simulink model "sim_Motor_2kW_openloop_v3_delay"  (Simulink 7.9)
settings: Solver=ode45  StartTime=0.0  StopTime=0.08  RelTol=1e-3
libraries: powerlib x7, simulink_extras x2
settings Model: Creator=Kun Zhang  LastModifiedBy=LYN
settings SolverCC: AutoInsertRateTranBlk=on
settings DebuggingCC: MultiTaskDSMMsg=warning  MultiTaskCondExecSysMsg=none  StrictBusMsg=None
settings RTWCC: IncludeERTFirstTime=on
settings GRTTargetCC: CombineOutputUpdateFcns=off  GRTInterface=on

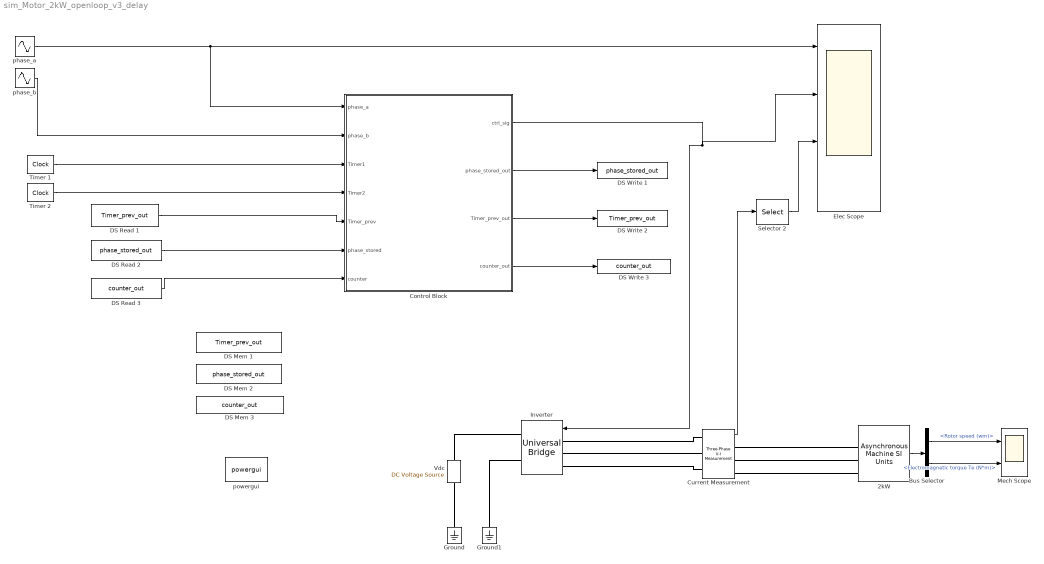
== system sim_Motor_2kW_openloop_v3_delay ==
  2kW : powerlib/Machines/Asynchronous Machine SI Units  PresetModel=No  MechanicalLoad=Torque Tm  ShowDetailedParameters=on  RotorType=Squirrel-cage  ReferenceFrame=Rotor  NominalParameters=[ 2000, 220, 50 ]  Stator=[ 1.115 0.005974]  Rotor=[ 1.083 0.005974]  Cage1=[ 0.022 0.226/377]  Cage2=[ 0.022 0.226/377]  Lm=0.2037  Mechanical=[0.02 0.005752 2]  PolePairs=2  InitialConditions=[1 0 0 0 0 0 0 0]  Units=SI  LoadFlowParameters=1492000  SimulateSaturation=off  Saturation=[14.03593122, 27.81365428, 53.79336849, 72.68890987, 97.98006896, 148.6815601, 215.7428561, 302.9841135, 428.7778367 ; 230, 322, 414, 460, 506, 552, 598, 644, 690]  TsPowergui=0  TsBlock=-1  IterativeModel=Forward Euler  Pmec=0
  Bus Selector : BusSelector  OutputSignals=Mechanical.Rotor speed (wm),Mechanical.Electromagnetic torque Te (N*m)
  Control Block : MATLAB Function  TreatAsAtomicUnit=on
  Current Measurement : powerlib/Measurements/Three-Phase V-I Measurement  VoltageMeasurement=no  SetLabelV=off  LabelV=Vabc  Vpu=off  VpuLL=off  CurrentMeasurement=yes  SetLabelI=off  LabelI=Iabc  Ipu=off  Pbase=100e6  Vbase=500e3  OutputType=Complex  PhasorSimulation=off  PSBequivalent=0
  DS Mem 1 : DataStoreMemory  DataStoreName=Timer_prev_out  ReadBeforeWriteMsg=warning  WriteAfterWriteMsg=warning  WriteAfterReadMsg=warning  InitialValue=[0;0]
  DS Mem 2 : DataStoreMemory  DataStoreName=phase_stored_out  ReadBeforeWriteMsg=warning  WriteAfterWriteMsg=warning  WriteAfterReadMsg=warning  InitialValue=[0;0;0]
  DS Mem 3 : DataStoreMemory  DataStoreName=counter_out  ReadBeforeWriteMsg=warning  WriteAfterWriteMsg=warning  WriteAfterReadMsg=warning
  DS Read 1 : DataStoreRead  DataStoreName=Timer_prev_out
  DS Read 2 : DataStoreRead  DataStoreName=phase_stored_out
  DS Read 3 : DataStoreRead  DataStoreName=counter_out
  DS Write 1 : DataStoreWrite  DataStoreName=phase_stored_out
  DS Write 2 : DataStoreWrite  DataStoreName=Timer_prev_out
  DS Write 3 : DataStoreWrite  DataStoreName=counter_out
  "Elec Scope " : Scope  NumInputPorts=4
      settings: TimeRange=0.00032  YMin=0.83~0~-3.25~-1  YMax=0.98~1~-1.25~1  SaveName=motor_2kW_elec
  Ground : powerlib/Elements/Ground  LConnTagsString=a
  Ground1 : powerlib/Elements/Ground  LConnTagsString=a
  Inverter : powerlib/Power Electronics/Universal Bridge  Arms=3  SnubberResistance=5000  SnubberCapacitance=inf  Device=IGBT / Diodes  Ron=1e-3  Lon=0  ForwardVoltages="[  0  0  ]"  ForwardVoltage=0  GTOparameters=[ 10e-6 , 20e-6 ]  IGBTparameters=[ 1e-6 , 1e-6 ]  Measurements=None  Measurements_2=None  converterType=Rectifier
  Mech Scope : Scope  NumInputPorts=2
      settings: TimeRange=0.01  YMin=-1~-5  YMax=1~5  SaveName=motor_2kW_mech
  Selector 2 : Selector  InputPortWidth=3  IndexOptions=Index vector (dialog)  Indices=[1]  OutputSizes=1
  Timer 1 : simulink_extras/Flip Flops/Clock  period=1/5000
  Timer 2 : simulink_extras/Flip Flops/Clock  period=1/(5000*100)
  Vdc : powerlib/Electrical Sources/DC Voltage Source  Amplitude=400  Measurements=None
  "phase_a " : Sin  Frequency=2*pi*300  SampleTime=1/(100*1000)
  "phase_b " : Sin  Frequency=2*pi*300  Phase=2*pi/3  SampleTime=1/(100*1000)
  powergui : powerlib/powergui  Priority=1  SimulationMode=Discrete  SolverType=Tustin  SampleTime=1e-6  frequency=60  SPID=off  DisableSnubberDevices=off  DisableRonSwitches=off  DisableVfSwitches=off  SwTol=0  Interpol=off  DisplayEquations=off  FunctionMessages=off  frequencyindice=50  Pbase=100e6  ErrMax=1e-4  Iterations=50  UnitsV=kV  UnitsW=MW  echomessages=off  HookPort=off  EnableUseOfTLC=off  x0status=blocks  RestoreLinks=warning  ResistiveCurrentMeasurement=off  Ylog=off  Xlog=on  ShowGrid=off  save=off  variable=ZData  structure=motor_2kW_elec  ZoomFFT=off  StartTime=0.0  cycles=1  DisplayStyle=1  fundamental=60  FreqAxis=off  MaxFrequency=1000  frequencyindicesteady=1  display=off  methode=off
  wires:
  2kW/1 -> Bus Selector/1
  Bus Selector/1 -> Mech Scope/1  "<Rotor speed (wm)>"
  Bus Selector/2 -> Mech Scope/2  "<Electromagnetic torque Te (N*m)>"
  "phase_b "/1 -> Control Block/2(phase_b)
  "phase_a "/1 -> Control Block/1(phase_a), "Elec Scope "/1
  Control Block/1(ctrl_sig) -> Inverter/1, "Elec Scope "/2
  DS Read 1/1 -> Control Block/5(Timer_prev)
  Control Block/3(Timer_prev_out) -> DS Write 2/1
  DS Read 2/1 -> Control Block/6(phase_stored)
  Control Block/2(phase_stored_out) -> DS Write 1/1
  DS Read 3/1 -> Control Block/7(counter)
  Control Block/4(counter_out) -> DS Write 3/1
  Timer 2/1 -> Control Block/4(Timer2)
  Timer 1/1 -> Control Block/3(Timer1)
  Current Measurement/1 -> Selector 2/1
  Selector 2/1 -> "Elec Scope "/3
  connections:
  Ground/LConn1 -- Vdc/LConn1
  Vdc/RConn1 -- Inverter/RConn1
  Inverter/RConn2 -- Ground1/LConn1
  Inverter/LConn1 -- Current Measurement/LConn1
  Inverter/LConn2 -- Current Measurement/LConn2
  Current Measurement/RConn1 -- 2kW/LConn1
  Current Measurement/RConn2 -- 2kW/LConn2
  Current Measurement/RConn3 -- 2kW/LConn3
  Inverter/LConn3 -- Current Measurement/LConn3

== matlab function Control Block ==
  data: phase_a input double; ctrl_sig output double; phase_stored_out output double; phase_b input double; Timer1 input double; Timer2 input double; Timer_prev input double; phase_stored input double; Timer_prev_out output double; counter input double; counter_out output double
function [ctrl_sig,phase_stored_out,Timer_prev_out,counter_out] = ctrl_blk_v3(phase_a,phase_b,Timer1,Timer2,Timer_prev,phase_stored,counter)
%%%%%%%%%%%%%%%%%%%%%%%%%%%%%%%%%%%%%%%%%%%%%%%%%%%%%%%%%%%%%%%%%%%%%%%%%%%%%%%%%%%%%%%%%%%%%%%%%%%%%%%%%%%%%%%%%%%%%%%%%%%%%%%%%%%%%%%%%%%%%%%%%%%%%%%%%%%%%%%%%
%                                                                                                                                                               %
%           The aim is to:                                                                                                                                      %                                                           
%           generate 3-phase PWM waveform using principle of PWM in simulink                                                                                    %                      
%           Version 1, written by Kun Zhang                                                                                                                     %                                          
%                                                                                                                                                               %
%           The input parameters are                                                                                                                            %                                               
%           phase_a: reference signal a                                                                                                                         %                              
%           phase_b: reference signal b                                                                                                                         %         
%           t: running time                                                                                                                                     %                      
%           Timer1: input clock signal determines the period of PWM                                                                                             %                                             
%           Timer2: input clock signal, 100 times greater than Timer 1                                                                                          %
%           ton: on period                                                                                                                                      %
%           tstart: start time                                                                                                                                  %
%                                                                                                                                                               %
%%%%%%%%%%%%%%%%%%%%%%%%%%%%%%%%%%%%%%%%%%%%%%%%%%%%%%%%%%%%%%%%%%%%%%%%%%%%%%%%%%%%%%%%%%%%%%%%%%%%%%%%%%%%%%%%%%%%%%%%%%%%%%%%%%%%%%%%%%%%%%%%%%%%%%%%%%%%%%%%%
%space reserved for gloabal variables declaration


%%%%%%%%%%%%%%%%%%%%%%%%%%%%%%%%%%%%%%%%%%%%%%%%%%%%%%%%%%%%%%%%%%%%%%%%%%%%%%%%%%%%%%%%%%%%%%%%%%%%%%%%%%%%%%%%%%%%%%%%%%%%%%%%%%%%%%%%%%%%%%%%%%%%%%%%%%%%%%%%%
REF_AMP= 1;                                                                 %magnitude of reference
DEAD_TIME= 10;                                                             	%dead time in ticks of Timer2
Timer_Ratio= 100;                                                           %the ratio of Timer1 to Timer2
phase_c= -phase_a-phase_b;                                             
phase_a= floor((phase_a+REF_AMP)*Timer_Ratio/2);                            %shift and scale phase a so that it ranges from 0 to 100 and digitalize
phase_b= floor((phase_b+REF_AMP)*Timer_Ratio/2);
phase_c= floor((phase_c+REF_AMP)*Timer_Ratio/2);   


%%%%%%%%%%%%%%%%%%%%%%%%%%%%%%%%%%%%%%%%%%%%%%%%%%%%%%%%%%%%%%%%%%%%%%%%%%%%%%%%%%%%%%%%%%%%%%%%%%%%%%%%%%%%%%%%%%%%%%%%%%%%%%%%%%%%%%%%%%%%%%%%%%%%%%%%%%%%%%%%%
if      Timer_prev(1)<0.2 && Timer1>0.8                                   	%if positive edge for Timer1
                phase_stored_out= floor([phase_a;phase_b;phase_c])
                counter= 0;                                                 %reset counter
else
                phase_stored_out= phase_stored;                             %if not postive edge, phase stored remains
end

if      Timer_prev(2)<0.2 && Timer2>0.8                                     %if positive edge of Timer2
                counter= counter+1;                                         %counter ranging from 0 to 100
end

%leg 1
if      counter<phase_stored(1)                                             %if counter is less or equal to stored phase
                pwm_1= 0;               pwm_2= 1;        
elseif  counter-phase_stored(1)<DEAD_TIME                                   %if counter is equal or greater than stored phase but the difference is less than dead time
                pwm_1= 0;               pwm_2= 0;
else
                pwm_1= 1;               pwm_2= 0;                           
end

%leg 2       
if      counter<phase_stored(2)                                         
                pwm_3= 0;               pwm_4= 1;        
elseif  counter-phase_stored(2)<DEAD_TIME
                pwm_3= 0;               pwm_4= 0;
else
                pwm_3= 1;               pwm_4= 0;
end

%leg 3       
if      counter+1<phase_stored(3)                                     
                pwm_5= 0;               pwm_6= 1;        
elseif  counter-phase_stored(3)<DEAD_TIME
                pwm_5= 0;               pwm_6= 0;
else
                pwm_5= 1;               pwm_6= 0;
end

if      counter<DEAD_TIME                                                   %initially, pwm 1->0, delay for 5 ticks (at the rate of Timer2)                                                     
                pwm_1= 0;               pwm_2= 0;
                pwm_3= 0;               pwm_5= 0;                
                pwm_5= 0;               pwm_6= 0;                
end


%%%%%%%%%%%%%%%%%%%%%%%%%%%%%%%%%%%%%%%%%%%%%%%%%%%%%%%%%%%%%%%%%%%%%%%%%%%%%%%%%%%%%%%%%%%%%%%%%%%%%%%%%%%%%%%%%%%%%%%%%%%%%%%%%%%%%%%%%%%%%%%%%%%%%%%%%%%%%%%%%
ctrl_sig= [pwm_1 pwm_2 pwm_3 pwm_4 pwm_5 pwm_6]';                           %six phase PWM
Timer_prev_out= [Timer1 Timer2]';
counter_out= counter;
